simulink subsystem "internal_cell_givens"  (R2020b)
settings: Solver=VariableStepAuto  StartTime=0.0  StopTime=10.0  RelTol=1e-3
values from neighbouring files (symbols this model uses):
  lambda = 0.995    [env_sim_setup.m]
  sigma = 1e-6    (= 1e-06)    [env_sim_setup.m]
settings Model: Creator=johngentile  LastModifiedBy=jgentile

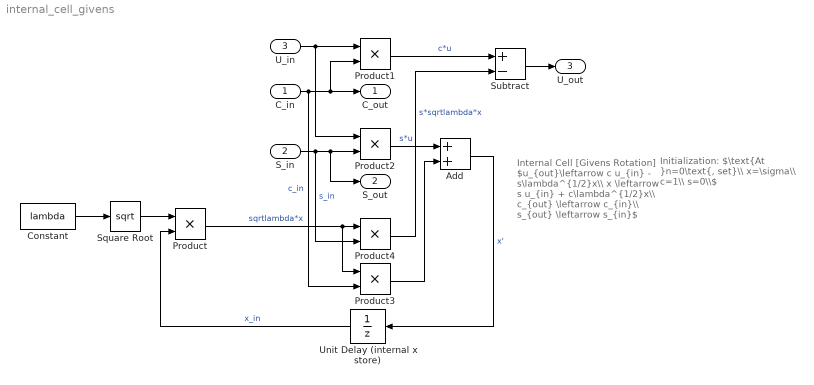
== system internal_cell_givens ==
  note: Internal Cell [Givens Rotation]
      | $u_{out}\leftarrow c u_{in} - s\lambda^{1/2}x\\ x \leftarrow s u_{in} + c\lambda^{1/2}x\\ c_{out} \leftarrow c_{in}\\ s_{out} \leftarrow s_{in}$
  note: Initialization:
      | $\text{At }n=0\text{, set}\\ x=\sigma\\ c=1\\ s=0\\$
  C_in : Inport
  S_in : Inport  Port=2
  U_in : Inport  Port=3
  Add : Sum
  Constant : Constant  Value=lambda
  Product{,1..4} (5 alike) : Product
  Square Root : Sqrt  SaturateOnIntegerOverflow=on
  Subtract : Sum  Inputs=+-
  Unit Delay (internal x store) : UnitDelay  InitialCondition=sigma  SampleTime=-1  HasFrameUpgradeWarning=on
  C_out : Outport
  S_out : Outport  Port=2
  U_out : Outport  Port=3
  wires:
  C_in/1 -> Product3/2, Product1/2, C_out/1  "c_in"
  Product/1 -> Product4/1, Product3/1  "sqrtlambda*x"
  S_in/1 -> Product4/2, Product2/2, S_out/1  "s_in"
  U_in/1 -> Product2/1, Product1/1
  Unit Delay (internal x store)/1 -> Product/2  "x_in"
  Add/1 -> Unit Delay (internal x store)/1  "x'"
  Product1/1 -> Subtract/1  "c*u"
  Subtract/1 -> U_out/1
  Product2/1 -> Add/1  "s*u"
  Product4/1 -> Subtract/2  "s*sqrtlambda*x"
  Product3/1 -> Add/2
  Constant/1 -> Square Root/1
  Square Root/1 -> Product/1
